simulink model "IMC"  (R2018b)
settings: Solver=VariableStepAuto  StartTime=0.0  StopTime=10.0  RelTol=1e-3
settings Model: Creator=Abdou  LastModifiedBy=Abdou

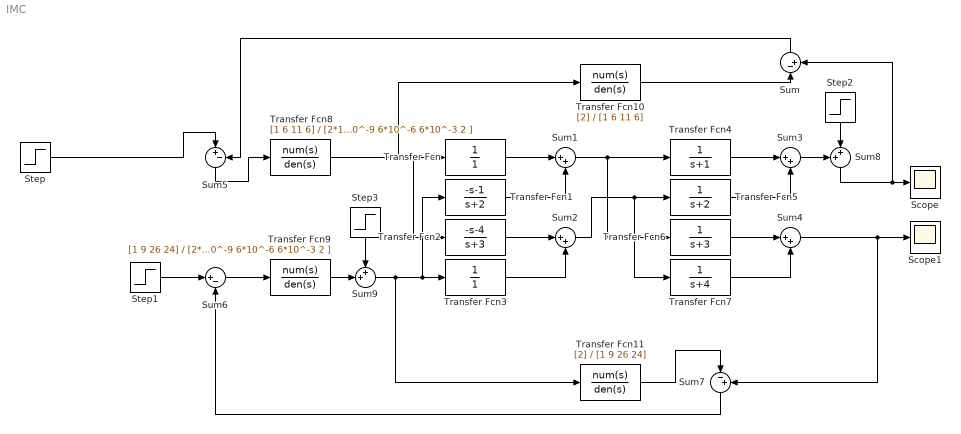
== system IMC ==
  Scope : Scope
  Scope1 : Scope
  Step : Step  SampleTime=0
  Step1 : Step  SampleTime=0
  Step2 : Step  Time=3  SampleTime=0
  Step3 : Step  Time=3  SampleTime=0
  Sum : Sum  Inputs=|-+
  Sum{1..4} (4 alike) : Sum  Inputs=|++
  Sum5 : Sum  Inputs=|+-
  Sum6 : Sum  Inputs=|+-
  Sum7 : Sum  Inputs=|-+
  Sum8 : Sum  Inputs=++|
  Sum9 : Sum  Inputs=++|
  Transfer Fcn : TransferFcn  Denominator=[1]
  Transfer Fcn1 : TransferFcn  Numerator=[-1 -1]  Denominator=[1 2]
  Transfer Fcn10 : TransferFcn  Numerator=[2]  Denominator=[1 6 11 6]
  Transfer Fcn11 : TransferFcn  Numerator=[2]  Denominator=[1 9 26 24]
  Transfer Fcn2 : TransferFcn  Numerator=[-1 -4]  Denominator=[1 3]
  Transfer Fcn3 : TransferFcn  Denominator=[1]
  Transfer Fcn4 : TransferFcn  Denominator=[1 1]
  Transfer Fcn5 : TransferFcn  Denominator=[1 2]
  Transfer Fcn6 : TransferFcn  Denominator=[1 3]
  Transfer Fcn7 : TransferFcn  Denominator=[1 4]
  Transfer Fcn8 : TransferFcn  Numerator=[1 6 11 6]  Denominator=[2*10^-9 6*10^-6 6*10^-3 2 ]
  Transfer Fcn9 : TransferFcn  Numerator=[1 9 26 24]  Denominator=[2*10^-9 6*10^-6 6*10^-3 2 ]
  wires:
  Transfer Fcn/1 -> Sum1/1
  Transfer Fcn1/1 -> Sum1/2
  Transfer Fcn2/1 -> Sum2/1
  Transfer Fcn3/1 -> Sum2/2
  Sum1/1 -> Transfer Fcn6/1, Transfer Fcn4/1
  Sum2/1 -> Transfer Fcn7/1, Transfer Fcn5/1
  Transfer Fcn4/1 -> Sum3/1
  Transfer Fcn5/1 -> Sum3/2
  Transfer Fcn6/1 -> Sum4/1
  Transfer Fcn7/1 -> Sum4/2
  Sum4/1 -> Scope1/1, Sum7/2
  Sum5/1 -> Transfer Fcn8/1
  Step/1 -> Sum5/1
  Step1/1 -> Sum6/1
  Transfer Fcn8/1 -> Transfer Fcn10/1, Transfer Fcn2/1, Transfer Fcn/1
  Sum6/1 -> Transfer Fcn9/1
  Transfer Fcn10/1 -> Sum/1
  Sum/1 -> Sum5/2
  Transfer Fcn11/1 -> Sum7/1
  Sum7/1 -> Sum6/2
  Sum3/1 -> Sum8/1
  Sum8/1 -> Sum/2, Scope/1
  Step2/1 -> Sum8/2
  Transfer Fcn9/1 -> Sum9/2
  Sum9/1 -> Transfer Fcn11/1, Transfer Fcn1/1, Transfer Fcn3/1
  Step3/1 -> Sum9/1
